simulink model "matrix7"  (R2018b)
settings: Solver=VariableStepAuto  StartTime=0.0  StopTime=3  RelTol=1e-7
model workspace (MAT data in the model file):
  A1 = 0.212
  A2 = 0.0033
  AMP1 = 0.209333333333
  AMP2 = 0.0330526315789
  B1 = 0.311
  B2 = 0.0075
  C1 = 0.1
  C2 = 0.0084
  Ce1 = 0.27
  Ce2 = 0.12
  Cm1 = 0.36
  Cm2 = 0.12
  D1 = 0.1
  D2 = 0.001
  E1 = 0.1
  E2 = 0.001
  F1 = 0.1
  F2 = 0.001
  Jdrv1 = 7.5e-06
  Jdrv2 = 2.51e-06
  Kf1 = 0.9
  Kf2 = 0.9
  L1 = 0.032
  L2 = 0.0194
  R1 = 0.32
  R2 = 0.485
  RAMP = 0.209333333333
  T1 = 0.05
  T2 = 0.0001
  Tpwm = 6.25e-05
  Umax = 27
  Xc2 = 0
  Yc2 = 0.0148
  a = 0
  b = -2.09439510239
  c = 2.09439510239
  dt1 = 0.6
  dt2 = 0.6
  dx1 = 3.14
  dx2 = 1.57
  g = 9.81
  m2 = 1.13085
  omega1 = 1.005
  omega2 = 6.28
  poles = 8
libraries: simulink x1
(part 2 of 2)

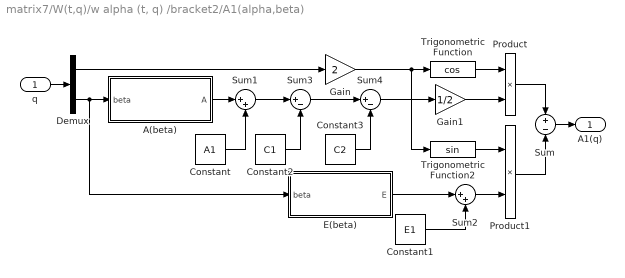
== system matrix7/W(t,q)/w alpha (t, q) /bracket2/A1(alpha,beta) ==
  q : Inport
  A(beta) : Subsystem
  Constant : Constant  Value=A1
  Constant1 : Constant  Value=E1
  Constant2 : Constant  Value=C1
  Constant3 : Constant  Value=C2
  Demux : Demux  Outputs=2
  E(beta) : Subsystem
  Gain : Gain  Gain=2
  Gain1 : Gain  Gain=1/2
  Product : Product
  Product1 : Product
  Sum : Sum  Inputs=+-
  Sum1 : Sum  Inputs=|++
  Sum2 : Sum  Inputs=|++
  Sum3 : Sum  Inputs=|+-
  Sum4 : Sum  Inputs=|+-
  Trigonometric Function : Trigonometry  Operator=cos
  Trigonometric Function2 : Trigonometry
  A1(q) : Outport
  wires:
  Trigonometric Function2/1 -> Product1/1
  Product1/1 -> Sum/2
  Trigonometric Function/1 -> Product/1
  Product/1 -> Sum/1
  Demux/1 -> Gain/1
  Sum/1 -> A1(q)/1
  A(beta)/1(A) -> Sum1/1
  Constant/1 -> Sum1/2
  Sum1/1 -> Sum3/1
  Demux/2 -> E(beta)/1(beta), A(beta)/1(beta)
  E(beta)/1(E) -> Sum2/1
  Constant1/1 -> Sum2/2
  Sum2/1 -> Product1/2
  q/1 -> Demux/1
  Sum3/1 -> Sum4/1
  Sum4/1 -> Gain1/1
  Constant2/1 -> Sum3/2
  Constant3/1 -> Sum4/2
  Gain/1 -> Trigonometric Function2/1, Trigonometric Function/1
  Gain1/1 -> Product/2

== system matrix7/W(t,q)/w alpha (t, q) /bracket2/D(alpha,beta) ==
  q : Inport
  Constant : Constant  Value=F1
  Constant1 : Constant  Value=D1
  D(beta) : Subsystem
  Demux : Demux  Outputs=2
  F(beta) : Subsystem
  Product : Product
  Product1 : Product
  Sum : Sum  Inputs=-+
  Sum1 : Sum  Inputs=|++
  Sum2 : Sum  Inputs=|++
  Trigonometric Function : Trigonometry
  Trigonometric Function2 : Trigonometry  Operator=cos
  D(q) : Outport
  wires:
  Trigonometric Function2/1 -> Product1/1
  Product1/1 -> Sum/2
  Trigonometric Function/1 -> Product/1
  Product/1 -> Sum/1
  Demux/1 -> Trigonometric Function2/1, Trigonometric Function/1
  Sum/1 -> D(q)/1
  F(beta)/1(F) -> Sum1/1
  Constant/1 -> Sum1/2
  Sum1/1 -> Product/2
  Demux/2 -> D(beta)/1(beta), F(beta)/1(beta)
  D(beta)/1(D) -> Sum2/1
  Constant1/1 -> Sum2/2
  Sum2/1 -> Product1/2
  q/1 -> Demux/1

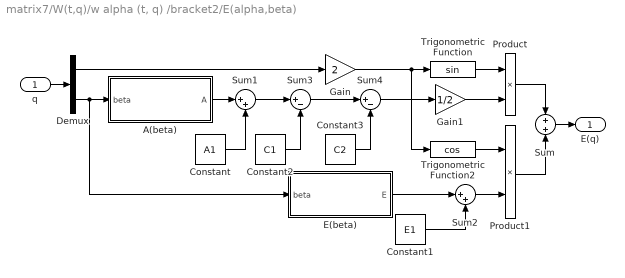
== system matrix7/W(t,q)/w alpha (t, q) /bracket2/E(alpha,beta) ==
  q : Inport
  A(beta) : Subsystem
  Constant : Constant  Value=A1
  Constant1 : Constant  Value=E1
  Constant2 : Constant  Value=C1
  Constant3 : Constant  Value=C2
  Demux : Demux  Outputs=2
  E(beta) : Subsystem
  Gain : Gain  Gain=2
  Gain1 : Gain  Gain=1/2
  Product : Product
  Product1 : Product
  Sum : Sum
  Sum1 : Sum  Inputs=|++
  Sum2 : Sum  Inputs=|++
  Sum3 : Sum  Inputs=|+-
  Sum4 : Sum  Inputs=|+-
  Trigonometric Function : Trigonometry
  Trigonometric Function2 : Trigonometry  Operator=cos
  E(q) : Outport
  wires:
  Trigonometric Function2/1 -> Product1/1
  Product1/1 -> Sum/2
  Trigonometric Function/1 -> Product/1
  Product/1 -> Sum/1
  Demux/1 -> Gain/1
  Sum/1 -> E(q)/1
  A(beta)/1(A) -> Sum1/1
  Constant/1 -> Sum1/2
  Sum1/1 -> Sum3/1
  Demux/2 -> E(beta)/1(beta), A(beta)/1(beta)
  E(beta)/1(E) -> Sum2/1
  Constant1/1 -> Sum2/2
  Sum2/1 -> Product1/2
  q/1 -> Demux/1
  Sum3/1 -> Sum4/1
  Sum4/1 -> Gain1/1
  Constant2/1 -> Sum3/2
  Constant3/1 -> Sum4/2
  Gain/1 -> Trigonometric Function2/1, Trigonometric Function/1
  Gain1/1 -> Product/2

== system matrix7/W(t,q)/w alpha (t, q) /bracket2/F(alpha,beta) ==
  q : Inport
  Constant : Constant  Value=F1
  Constant1 : Constant  Value=D1
  D(beta) : Subsystem
  Demux : Demux  Outputs=2
  F(beta) : Subsystem
  Product : Product
  Product1 : Product
  Sum : Sum
  Sum1 : Sum  Inputs=|++
  Sum2 : Sum  Inputs=|++
  Trigonometric Function : Trigonometry  Operator=cos
  Trigonometric Function2 : Trigonometry
  F(q) : Outport
  wires:
  Trigonometric Function2/1 -> Product1/1
  Product1/1 -> Sum/2
  Trigonometric Function/1 -> Product/1
  Product/1 -> Sum/1
  Demux/1 -> Trigonometric Function2/1, Trigonometric Function/1
  Sum/1 -> F(q)/1
  F(beta)/1(F) -> Sum1/1
  Constant/1 -> Sum1/2
  Sum1/1 -> Product/2
  Demux/2 -> D(beta)/1(beta), F(beta)/1(beta)
  D(beta)/1(D) -> Sum2/1
  Constant1/1 -> Sum2/2
  Sum2/1 -> Product1/2
  q/1 -> Demux/1

== system matrix7/W(t,q)/w beta (t, q)/bracket1/D(beta) ==
  beta : Inport
  Gain : Gain  Gain=D2
  Gain2 : Gain  Gain=E2
  Sum : Sum
  Trigonometric Function : Trigonometry  Operator=cos
  Trigonometric Function2 : Trigonometry
  D : Outport
  wires:
  Gain2/1 -> Sum/2
  Sum/1 -> D/1
  Gain/1 -> Sum/1
  beta/1 -> Trigonometric Function/1, Trigonometric Function2/1
  Trigonometric Function2/1 -> Gain2/1
  Trigonometric Function/1 -> Gain/1

== system matrix7/W(t,q)/w beta (t, q)/bracket1/E(beta) ==
  beta : Inport
  Gain : Gain  Gain=E2
  Gain2 : Gain  Gain=D2
  Sum : Sum  Inputs=+-
  Trigonometric Function : Trigonometry  Operator=cos
  Trigonometric Function2 : Trigonometry
  E : Outport
  wires:
  Gain2/1 -> Sum/2
  Sum/1 -> E/1
  Gain/1 -> Sum/1
  beta/1 -> Trigonometric Function/1, Trigonometric Function2/1
  Trigonometric Function2/1 -> Gain2/1
  Trigonometric Function/1 -> Gain/1

== system matrix7/W(t,q)/w beta (t, q)/bracket1/E(beta)1 ==
  beta : Inport
  Gain : Gain  Gain=E2
  Gain2 : Gain  Gain=D2
  Sum : Sum  Inputs=+-
  Trigonometric Function : Trigonometry  Operator=cos
  Trigonometric Function2 : Trigonometry
  E : Outport
  wires:
  Gain2/1 -> Sum/2
  Sum/1 -> E/1
  Gain/1 -> Sum/1
  beta/1 -> Trigonometric Function/1, Trigonometric Function2/1
  Trigonometric Function2/1 -> Gain2/1
  Trigonometric Function/1 -> Gain/1

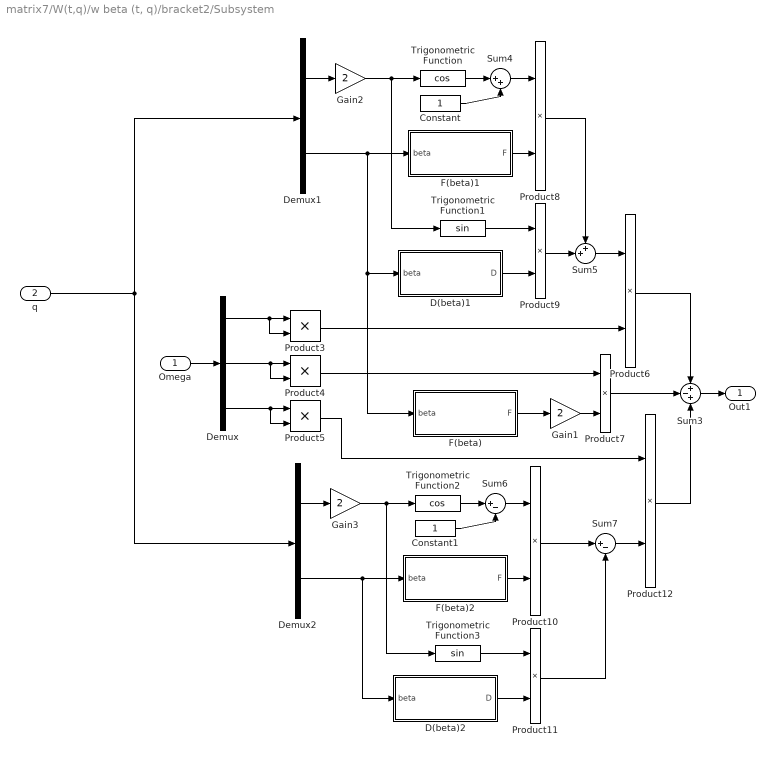
== system matrix7/W(t,q)/w beta (t, q)/bracket2/Subsystem ==
  Omega : Inport
  q : Inport  Port=2
  Constant : Constant
  Constant1 : Constant
  D(beta)1 : Subsystem
  D(beta)2 : Subsystem
  Demux : Demux  Outputs=3
  Demux1 : Demux  Outputs=2
  Demux2 : Demux  Outputs=2
  F(beta) : Subsystem
  F(beta)1 : Subsystem
  F(beta)2 : Subsystem
  Gain1 : Gain  Gain=2
  Gain2 : Gain  Gain=2
  Gain3 : Gain  Gain=2
  Product{3..12} (10 alike) : Product
  Sum3 : Sum  Inputs=+-+
  Sum4 : Sum  Inputs=|++
  Sum5 : Sum  Inputs=++|
  Sum6 : Sum  Inputs=|+-
  Sum7 : Sum  Inputs=|+-
  Trigonometric Function : Trigonometry  Operator=cos
  Trigonometric Function1 : Trigonometry
  Trigonometric Function2 : Trigonometry  Operator=cos
  Trigonometric Function3 : Trigonometry
  Out1 : Outport
  wires:
  Trigonometric Function/1 -> Sum4/1
  Constant1/1 -> Sum6/2
  Demux2/2 -> D(beta)2/1(beta), F(beta)2/1(beta)
  Product10/1 -> Sum7/1
  Demux2/1 -> Gain3/1
  F(beta)2/1(F) -> Product10/2
  Gain3/1 -> Trigonometric Function3/1, Trigonometric Function2/1
  Sum6/1 -> Product10/1
  Trigonometric Function3/1 -> Product11/1
  D(beta)2/1(D) -> Product11/2
  Product12/1 -> Sum3/3
  Sum7/1 -> Product12/2
  Trigonometric Function2/1 -> Sum6/1
  Product8/1 -> Sum5/1
  Product9/1 -> Sum5/2
  Demux1/2 -> F(beta)/1(beta), D(beta)1/1(beta), F(beta)1/1(beta)
  Product6/1 -> Sum3/1
  F(beta)1/1(F) -> Product8/2
  D(beta)1/1(D) -> Product9/2
  Constant/1 -> Sum4/2
  Gain2/1 -> Trigonometric Function1/1, Trigonometric Function/1
  F(beta)/1(F) -> Gain1/1
  Product4/1 -> Product7/1
  Gain1/1 -> Product7/2
  Product3/1 -> Product6/2
  Product7/1 -> Sum3/2
  Product11/1 -> Sum7/2
  Demux1/1 -> Gain2/1
  Product5/1 -> Product12/1
  Trigonometric Function1/1 -> Product9/1
  Sum4/1 -> Product8/1
  Omega/1 -> Demux/1
  Demux/1 -> Product3/2, Product3/1
  Sum5/1 -> Product6/1
  Demux/2 -> Product4/2, Product4/1
  Demux/3 -> Product5/2, Product5/1
  q/1 -> Demux1/1, Demux2/1
  Sum3/1 -> Out1/1

== system matrix7/W(t,q)/w beta (t, q)/bracket2/Subsystem1 ==
  q : Inport
  omega x omega y : Inport  Port=2
  A2(beta) : Subsystem
  Demux1 : Demux  Outputs=2
  E(beta) : Subsystem
  Gain1 : Gain  Gain=2
  Product : Product
  Product1 : Product
  Product3 : Product
  Sum : Sum  Inputs=+-
  Trigonometric Function : Trigonometry  Operator=cos
  Trigonometric Function1 : Trigonometry
  Out1 : Outport
  wires:
  Trigonometric Function/1 -> Product/1
  Demux1/2 -> E(beta)/1(beta), A2(beta)/1(beta)
  Product/1 -> Sum/1
  Gain1/1 -> Product/2
  Trigonometric Function1/1 -> Product3/2
  A2(beta)/1(A2) -> Gain1/1
  Demux1/1 -> Trigonometric Function1/1, Trigonometric Function/1
  E(beta)/1(E) -> Product3/1
  Product3/1 -> Sum/2
  Sum/1 -> Product1/1
  Product1/1 -> Out1/1
  q/1 -> Demux1/1
  omega x omega y/1 -> Product1/2

== system matrix7/W(t,q)/w beta (t, q)/bracket2/Subsystem2 ==
  q : Inport
  omega x omega z : Inport  Port=2
  D(beta) : Subsystem
  Demux1 : Demux  Outputs=2
  F(beta) : Subsystem
  Gain : Gain  Gain=2
  Product : Product
  Product1 : Product
  Product3 : Product
  Sum : Sum  Inputs=+-
  Trigonometric Function : Trigonometry
  Trigonometric Function1 : Trigonometry  Operator=cos
  Out1 : Outport
  wires:
  omega x omega z/1 -> Product1/2
  q/1 -> Demux1/1
  Product1/1 -> Out1/1
  Sum/1 -> Product1/1
  Product3/1 -> Sum/2
  D(beta)/1(D) -> Product3/1
  Demux1/1 -> Gain/1
  Trigonometric Function1/1 -> Product3/2
  F(beta)/1(F) -> Product/2
  Product/1 -> Sum/1
  Trigonometric Function/1 -> Product/1
  Gain/1 -> Trigonometric Function/1, Trigonometric Function1/1
  Demux1/2 -> F(beta)/1(beta), D(beta)/1(beta)

== system matrix7/W(t,q)/w beta (t, q)/bracket2/Subsystem3 ==
  q : Inport
  omega y omega z : Inport  Port=2
  A2(beta) : Subsystem
  Demux1 : Demux  Outputs=2
  E(beta) : Subsystem
  Gain1 : Gain  Gain=2
  Product : Product
  Product1 : Product
  Product3 : Product
  Sum : Sum
  Trigonometric Function : Trigonometry  Operator=cos
  Trigonometric Function1 : Trigonometry
  Out1 : Outport
  wires:
  omega y omega z/1 -> Product1/2
  q/1 -> Demux1/1
  Product1/1 -> Out1/1
  Sum/1 -> Product1/1
  Product3/1 -> Sum/2
  Gain1/1 -> Product3/1
  Demux1/1 -> Trigonometric Function/1, Trigonometric Function1/1
  Trigonometric Function1/1 -> Product3/2
  E(beta)/1(E) -> Product/2
  Product/1 -> Sum/1
  Demux1/2 -> A2(beta)/1(beta), E(beta)/1(beta)
  Trigonometric Function/1 -> Product/1
  A2(beta)/1(A2) -> Gain1/1

== system matrix7/W(t,q)/w alpha (t, q) /bracket1/D(alpha,beta)/D(beta) ==
  beta : Inport
  Gain : Gain  Gain=D2
  Gain2 : Gain  Gain=E2
  Sum : Sum
  Trigonometric Function : Trigonometry  Operator=cos
  Trigonometric Function2 : Trigonometry
  D : Outport
  wires:
  Trigonometric Function/1 -> Gain/1
  Trigonometric Function2/1 -> Gain2/1
  beta/1 -> Trigonometric Function2/1, Trigonometric Function/1
  Gain/1 -> Sum/1
  Sum/1 -> D/1
  Gain2/1 -> Sum/2

== system matrix7/W(t,q)/w alpha (t, q) /bracket1/D(alpha,beta)/F(beta) ==
  beta : Inport
  Gain : Gain  Gain=F2
  Gain1 : Gain  Gain=2
  Gain2 : Gain  Gain=(A2-B2)/2
  Sum : Sum  Inputs=+-
  Trigonometric Function : Trigonometry  Operator=cos
  Trigonometric Function2 : Trigonometry
  F : Outport
  wires:
  Trigonometric Function/1 -> Gain/1
  Trigonometric Function2/1 -> Gain2/1
  beta/1 -> Trigonometric Function/1, Gain1/1
  Gain/1 -> Sum/1
  Sum/1 -> F/1
  Gain2/1 -> Sum/2
  Gain1/1 -> Trigonometric Function2/1

== system matrix7/W(t,q)/w alpha (t, q) /bracket1/F(alpha,beta)/D(beta) ==
  beta : Inport
  Gain : Gain  Gain=D2
  Gain2 : Gain  Gain=E2
  Sum : Sum
  Trigonometric Function : Trigonometry  Operator=cos
  Trigonometric Function2 : Trigonometry
  D : Outport
  wires:
  Trigonometric Function/1 -> Gain/1
  Trigonometric Function2/1 -> Gain2/1
  beta/1 -> Trigonometric Function2/1, Trigonometric Function/1
  Gain/1 -> Sum/1
  Sum/1 -> D/1
  Gain2/1 -> Sum/2

== system matrix7/W(t,q)/w alpha (t, q) /bracket1/F(alpha,beta)/F(beta) ==
  beta : Inport
  Gain : Gain  Gain=F2
  Gain1 : Gain  Gain=2
  Gain2 : Gain  Gain=(A2-B2)/2
  Sum : Sum  Inputs=+-
  Trigonometric Function : Trigonometry  Operator=cos
  Trigonometric Function2 : Trigonometry
  F : Outport
  wires:
  Trigonometric Function/1 -> Gain/1
  Trigonometric Function2/1 -> Gain2/1
  beta/1 -> Trigonometric Function/1, Gain1/1
  Gain/1 -> Sum/1
  Sum/1 -> F/1
  Gain2/1 -> Sum/2
  Gain1/1 -> Trigonometric Function2/1

== system matrix7/W(t,q)/w alpha (t, q) /bracket2/A1(alpha,beta)/A(beta) ==
  beta : Inport
  Constant : Constant  Value=2
  Constant1 : Constant  Value=2
  Gain : Gain  Gain=A2
  Gain1 : Gain  Gain=2
  Gain2 : Gain  Gain=F2
  Gain3 : Gain  Gain=B2
  Math Function : Math  Operator=pow  SaturateOnIntegerOverflow=on
  Math Function1 : Math  Operator=pow  SaturateOnIntegerOverflow=on
  Sum : Sum  Inputs=+++
  Trigonometric Function : Trigonometry  Operator=cos
  Trigonometric Function1 : Trigonometry
  Trigonometric Function2 : Trigonometry
  A : Outport
  wires:
  Trigonometric Function/1 -> Math Function/1
  Trigonometric Function2/1 -> Gain2/1
  Gain/1 -> Sum/1
  Sum/1 -> A/1
  Gain2/1 -> Sum/2
  Gain1/1 -> Trigonometric Function2/1
  Constant/1 -> Math Function/2
  Math Function/1 -> Gain/1
  Math Function1/1 -> Gain3/1
  Constant1/1 -> Math Function1/2
  beta/1 -> Trigonometric Function/1, Trigonometric Function1/1, Gain1/1
  Trigonometric Function1/1 -> Math Function1/1
  Gain3/1 -> Sum/3

== system matrix7/W(t,q)/w alpha (t, q) /bracket2/A1(alpha,beta)/E(beta) ==
  beta : Inport
  Gain : Gain  Gain=E2
  Gain2 : Gain  Gain=D2
  Sum : Sum  Inputs=+-
  Trigonometric Function : Trigonometry  Operator=cos
  Trigonometric Function2 : Trigonometry
  E : Outport
  wires:
  Trigonometric Function/1 -> Gain/1
  Trigonometric Function2/1 -> Gain2/1
  beta/1 -> Trigonometric Function2/1, Trigonometric Function/1
  Gain/1 -> Sum/1
  Sum/1 -> E/1
  Gain2/1 -> Sum/2

== system matrix7/W(t,q)/w alpha (t, q) /bracket2/D(alpha,beta)/D(beta) ==
  beta : Inport
  Gain : Gain  Gain=D2
  Gain2 : Gain  Gain=E2
  Sum : Sum
  Trigonometric Function : Trigonometry  Operator=cos
  Trigonometric Function2 : Trigonometry
  D : Outport
  wires:
  Trigonometric Function/1 -> Gain/1
  Trigonometric Function2/1 -> Gain2/1
  beta/1 -> Trigonometric Function2/1, Trigonometric Function/1
  Gain/1 -> Sum/1
  Sum/1 -> D/1
  Gain2/1 -> Sum/2

== system matrix7/W(t,q)/w alpha (t, q) /bracket2/D(alpha,beta)/F(beta) ==
  beta : Inport
  Gain : Gain  Gain=F2
  Gain1 : Gain  Gain=2
  Gain2 : Gain  Gain=(A2-B2)/2
  Sum : Sum  Inputs=+-
  Trigonometric Function : Trigonometry  Operator=cos
  Trigonometric Function2 : Trigonometry
  F : Outport
  wires:
  Trigonometric Function/1 -> Gain/1
  Trigonometric Function2/1 -> Gain2/1
  beta/1 -> Trigonometric Function/1, Gain1/1
  Gain/1 -> Sum/1
  Sum/1 -> F/1
  Gain2/1 -> Sum/2
  Gain1/1 -> Trigonometric Function2/1

== system matrix7/W(t,q)/w alpha (t, q) /bracket2/E(alpha,beta)/A(beta) ==
  beta : Inport
  Constant : Constant  Value=2
  Constant1 : Constant  Value=2
  Gain : Gain  Gain=A2
  Gain1 : Gain  Gain=2
  Gain2 : Gain  Gain=F2
  Gain3 : Gain  Gain=B2
  Math Function : Math  Operator=pow  SaturateOnIntegerOverflow=on
  Math Function1 : Math  Operator=pow  SaturateOnIntegerOverflow=on
  Sum : Sum  Inputs=+++
  Trigonometric Function : Trigonometry  Operator=cos
  Trigonometric Function1 : Trigonometry
  Trigonometric Function2 : Trigonometry
  A : Outport
  wires:
  Trigonometric Function/1 -> Math Function/1
  Trigonometric Function2/1 -> Gain2/1
  Gain/1 -> Sum/1
  Sum/1 -> A/1
  Gain2/1 -> Sum/2
  Gain1/1 -> Trigonometric Function2/1
  Constant/1 -> Math Function/2
  Math Function/1 -> Gain/1
  Math Function1/1 -> Gain3/1
  Constant1/1 -> Math Function1/2
  beta/1 -> Trigonometric Function/1, Trigonometric Function1/1, Gain1/1
  Trigonometric Function1/1 -> Math Function1/1
  Gain3/1 -> Sum/3

== system matrix7/W(t,q)/w alpha (t, q) /bracket2/E(alpha,beta)/E(beta) ==
  beta : Inport
  Gain : Gain  Gain=E2
  Gain2 : Gain  Gain=D2
  Sum : Sum  Inputs=+-
  Trigonometric Function : Trigonometry  Operator=cos
  Trigonometric Function2 : Trigonometry
  E : Outport
  wires:
  Trigonometric Function/1 -> Gain/1
  Trigonometric Function2/1 -> Gain2/1
  beta/1 -> Trigonometric Function2/1, Trigonometric Function/1
  Gain/1 -> Sum/1
  Sum/1 -> E/1
  Gain2/1 -> Sum/2

== system matrix7/W(t,q)/w alpha (t, q) /bracket2/F(alpha,beta)/D(beta) ==
  beta : Inport
  Gain : Gain  Gain=D2
  Gain2 : Gain  Gain=E2
  Sum : Sum
  Trigonometric Function : Trigonometry  Operator=cos
  Trigonometric Function2 : Trigonometry
  D : Outport
  wires:
  Trigonometric Function/1 -> Gain/1
  Trigonometric Function2/1 -> Gain2/1
  beta/1 -> Trigonometric Function2/1, Trigonometric Function/1
  Gain/1 -> Sum/1
  Sum/1 -> D/1
  Gain2/1 -> Sum/2

== system matrix7/W(t,q)/w alpha (t, q) /bracket2/F(alpha,beta)/F(beta) ==
  beta : Inport
  Gain : Gain  Gain=F2
  Gain1 : Gain  Gain=2
  Gain2 : Gain  Gain=(A2-B2)/2
  Sum : Sum  Inputs=+-
  Trigonometric Function : Trigonometry  Operator=cos
  Trigonometric Function2 : Trigonometry
  F : Outport
  wires:
  Trigonometric Function/1 -> Gain/1
  Trigonometric Function2/1 -> Gain2/1
  beta/1 -> Trigonometric Function/1, Gain1/1
  Gain/1 -> Sum/1
  Sum/1 -> F/1
  Gain2/1 -> Sum/2
  Gain1/1 -> Trigonometric Function2/1

== system matrix7/W(t,q)/w beta (t, q)/bracket2/Subsystem/D(beta)1 ==
  beta : Inport
  Gain : Gain  Gain=D2
  Gain2 : Gain  Gain=E2
  Sum : Sum
  Trigonometric Function : Trigonometry  Operator=cos
  Trigonometric Function2 : Trigonometry
  D : Outport
  wires:
  Trigonometric Function/1 -> Gain/1
  Trigonometric Function2/1 -> Gain2/1
  beta/1 -> Trigonometric Function2/1, Trigonometric Function/1
  Gain/1 -> Sum/1
  Sum/1 -> D/1
  Gain2/1 -> Sum/2

== system matrix7/W(t,q)/w beta (t, q)/bracket2/Subsystem/D(beta)2 ==
  beta : Inport
  Gain : Gain  Gain=D2
  Gain2 : Gain  Gain=E2
  Sum : Sum
  Trigonometric Function : Trigonometry  Operator=cos
  Trigonometric Function2 : Trigonometry
  D : Outport
  wires:
  Trigonometric Function/1 -> Gain/1
  Trigonometric Function2/1 -> Gain2/1
  beta/1 -> Trigonometric Function2/1, Trigonometric Function/1
  Gain/1 -> Sum/1
  Sum/1 -> D/1
  Gain2/1 -> Sum/2

== system matrix7/W(t,q)/w beta (t, q)/bracket2/Subsystem/F(beta) ==
  beta : Inport
  Gain : Gain  Gain=F2
  Gain1 : Gain  Gain=2
  Gain2 : Gain  Gain=(A2-B2)/2
  Sum : Sum  Inputs=+-
  Trigonometric Function : Trigonometry  Operator=cos
  Trigonometric Function2 : Trigonometry
  F : Outport
  wires:
  Gain1/1 -> Trigonometric Function2/1
  Gain2/1 -> Sum/2
  Sum/1 -> F/1
  Gain/1 -> Sum/1
  beta/1 -> Gain1/1, Trigonometric Function/1
  Trigonometric Function2/1 -> Gain2/1
  Trigonometric Function/1 -> Gain/1

== system matrix7/W(t,q)/w beta (t, q)/bracket2/Subsystem/F(beta)1 ==
  beta : Inport
  Gain : Gain  Gain=F2
  Gain1 : Gain  Gain=2
  Gain2 : Gain  Gain=(A2-B2)/2
  Sum : Sum  Inputs=+-
  Trigonometric Function : Trigonometry  Operator=cos
  Trigonometric Function2 : Trigonometry
  F : Outport
  wires:
  Trigonometric Function/1 -> Gain/1
  Trigonometric Function2/1 -> Gain2/1
  beta/1 -> Trigonometric Function/1, Gain1/1
  Gain/1 -> Sum/1
  Sum/1 -> F/1
  Gain2/1 -> Sum/2
  Gain1/1 -> Trigonometric Function2/1

== system matrix7/W(t,q)/w beta (t, q)/bracket2/Subsystem/F(beta)2 ==
  beta : Inport
  Gain : Gain  Gain=F2
  Gain1 : Gain  Gain=2
  Gain2 : Gain  Gain=(A2-B2)/2
  Sum : Sum  Inputs=+-
  Trigonometric Function : Trigonometry  Operator=cos
  Trigonometric Function2 : Trigonometry
  F : Outport
  wires:
  Trigonometric Function/1 -> Gain/1
  Trigonometric Function2/1 -> Gain2/1
  beta/1 -> Trigonometric Function/1, Gain1/1
  Gain/1 -> Sum/1
  Sum/1 -> F/1
  Gain2/1 -> Sum/2
  Gain1/1 -> Trigonometric Function2/1

== system matrix7/W(t,q)/w beta (t, q)/bracket2/Subsystem1/A2(beta) ==
  beta : Inport
  Gain : Gain  Gain=A2-B2
  Gain1 : Gain  Gain=2
  Gain2 : Gain  Gain=F2
  Gain3 : Gain  Gain=1/2
  Sum : Sum
  Trigonometric Function : Trigonometry  Operator=cos
  Trigonometric Function2 : Trigonometry
  A2 : Outport
  wires:
  Trigonometric Function/1 -> Gain/1
  Trigonometric Function2/1 -> Gain2/1
  beta/1 -> Gain1/1
  Gain/1 -> Gain3/1
  Sum/1 -> A2/1
  Gain2/1 -> Sum/2
  Gain1/1 -> Trigonometric Function/1, Trigonometric Function2/1
  Gain3/1 -> Sum/1

== system matrix7/W(t,q)/w beta (t, q)/bracket2/Subsystem1/E(beta) ==
  beta : Inport
  Gain : Gain  Gain=E2
  Gain2 : Gain  Gain=D2
  Sum : Sum  Inputs=+-
  Trigonometric Function : Trigonometry  Operator=cos
  Trigonometric Function2 : Trigonometry
  E : Outport
  wires:
  Gain2/1 -> Sum/2
  Sum/1 -> E/1
  Gain/1 -> Sum/1
  beta/1 -> Trigonometric Function/1, Trigonometric Function2/1
  Trigonometric Function2/1 -> Gain2/1
  Trigonometric Function/1 -> Gain/1

== system matrix7/W(t,q)/w beta (t, q)/bracket2/Subsystem2/D(beta) ==
  beta : Inport
  Gain : Gain  Gain=D2
  Gain2 : Gain  Gain=E2
  Sum : Sum
  Trigonometric Function : Trigonometry  Operator=cos
  Trigonometric Function2 : Trigonometry
  D : Outport
  wires:
  Gain2/1 -> Sum/2
  Sum/1 -> D/1
  Gain/1 -> Sum/1
  beta/1 -> Trigonometric Function/1, Trigonometric Function2/1
  Trigonometric Function2/1 -> Gain2/1
  Trigonometric Function/1 -> Gain/1

== system matrix7/W(t,q)/w beta (t, q)/bracket2/Subsystem2/F(beta) ==
  beta : Inport
  Gain : Gain  Gain=F2
  Gain1 : Gain  Gain=2
  Gain2 : Gain  Gain=(A2-B2)/2
  Sum : Sum  Inputs=+-
  Trigonometric Function : Trigonometry  Operator=cos
  Trigonometric Function2 : Trigonometry
  F : Outport
  wires:
  Trigonometric Function/1 -> Gain/1
  Trigonometric Function2/1 -> Gain2/1
  beta/1 -> Trigonometric Function/1, Gain1/1
  Gain/1 -> Sum/1
  Sum/1 -> F/1
  Gain2/1 -> Sum/2
  Gain1/1 -> Trigonometric Function2/1

== system matrix7/W(t,q)/w beta (t, q)/bracket2/Subsystem3/A2(beta) ==
  beta : Inport
  Gain : Gain  Gain=A2-B2
  Gain1 : Gain  Gain=2
  Gain2 : Gain  Gain=F2
  Gain3 : Gain  Gain=1/2
  Sum : Sum
  Trigonometric Function : Trigonometry  Operator=cos
  Trigonometric Function2 : Trigonometry
  A2 : Outport
  wires:
  Gain3/1 -> Sum/1
  Gain1/1 -> Trigonometric Function2/1, Trigonometric Function/1
  Gain2/1 -> Sum/2
  Sum/1 -> A2/1
  Gain/1 -> Gain3/1
  beta/1 -> Gain1/1
  Trigonometric Function2/1 -> Gain2/1
  Trigonometric Function/1 -> Gain/1

== system matrix7/W(t,q)/w beta (t, q)/bracket2/Subsystem3/E(beta) ==
  beta : Inport
  Gain : Gain  Gain=E2
  Gain2 : Gain  Gain=D2
  Sum : Sum  Inputs=+-
  Trigonometric Function : Trigonometry  Operator=cos
  Trigonometric Function2 : Trigonometry
  E : Outport
  wires:
  Trigonometric Function/1 -> Gain/1
  Trigonometric Function2/1 -> Gain2/1
  beta/1 -> Trigonometric Function2/1, Trigonometric Function/1
  Gain/1 -> Sum/1
  Sum/1 -> E/1
  Gain2/1 -> Sum/2

== matlab function matrix7/MATLAB Function ==
  data: u input; y output
function y = fcn(u)

y = inv(u);
